simulink model "pwpf_real_signal"  (R2021b)
settings: Solver=VariableStepAuto  StartTime=0.0  StopTime=t_sim  RelTol=1e-3
values from neighbouring files (symbols this model uses):
  Km_d = inputArg(2)    [cost_pwpf_dis.m]
  scale = length_real/(max(x)-min(x))    [model3d_maker.m]
  Tm_d = inputArg(1)    [cost_pwpf_dis.m]
  u_off = inputArg(4)    [cost_pwpf.m]    (also in cost_pwpf_dis.m)
  u_on = h+u_off    [cost_pwpf.m]    (also in cost_pwpf_dis.m)
undefined symbols (not defined in the file or in its folder): min_on_off_time, sample_time
settings Model: Creator=Mehdi  LastModifiedBy=Mehdi
settings SolverCC: ZeroCrossAlgorithm=Adaptive  AlgebraicLoopSolver=TrustRegion
settings DebuggingCC: IgnoredZcDiagnostic=none  SFMachineParentedDataDiag=warning

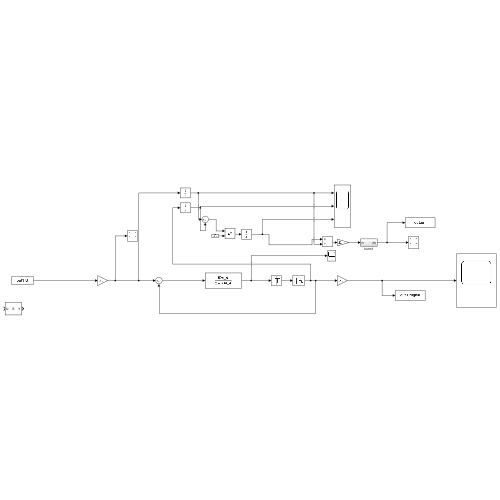
[thumbnail: Simulink's stored preview of the top-level diagram]
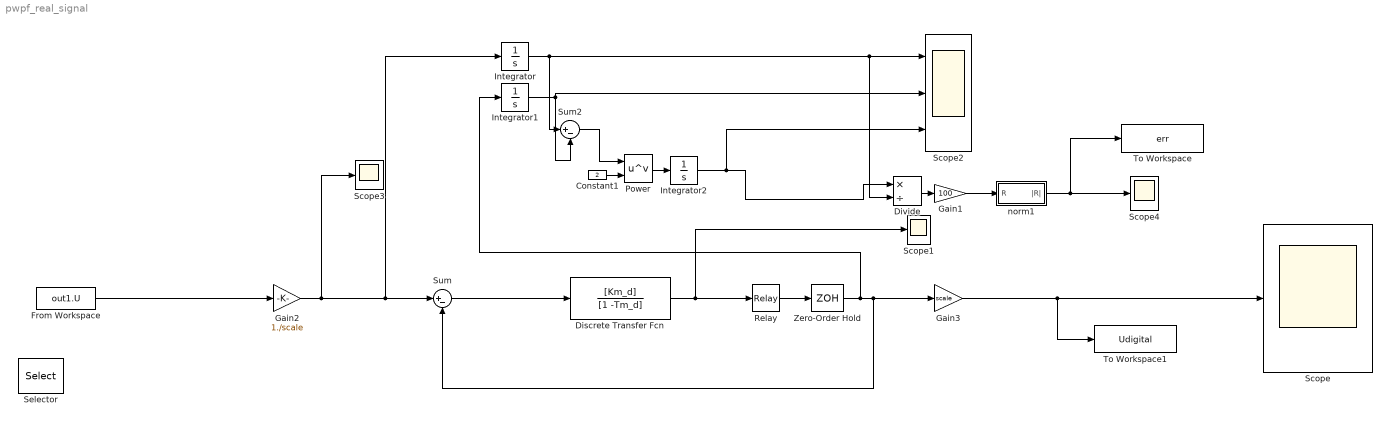
== system pwpf_real_signal ==
  Constant1 : Constant  Value=2  VectorParams1D=off
  Discrete Transfer Fcn : DiscreteTransferFcn  Numerator=[Km_d]  Denominator=[1 -Tm_d]  SampleTime=sample_time
  Divide : Product  Inputs=*/
  From Workspace : FromWorkspace  VariableName=out1.U
  Gain1 : Gain  Gain=100
  Gain2 : Gain  Gain=1./scale
  Gain3 : Gain  Gain=scale
  Integrator : Integrator
  Integrator1 : Integrator
  Integrator2 : Integrator
  Power : Math  Operator=pow  SaturateOnIntegerOverflow=on
  Relay : Relay  OnSwitchValue=u_on  OffSwitchValue=u_off  OnOutputValue=Thrust_digital
  Scope{,1,3..4} (4 alike) : Scope
  Scope2 : Scope  NumInputPorts=3
  Selector : Selector  InputPortWidth=30  IndexOptions=Index vector (dialog)  Indices=1  OutputSizes=1
  Sum : Sum  Inputs=|+-
  Sum2 : Sum  Inputs=|+-
  To Workspace : ToWorkspace  VariableName=err  SaveFormat=Timeseries  SampleTime=-1
      settings: MaxDataPoints=1
  To Workspace1 : ToWorkspace  VariableName=Udigital  SaveFormat=Timeseries  SampleTime=-1
  Zero-Order Hold : ZeroOrderHold  SampleTime=min_on_off_time
  norm1 : Subsystem
  wires:
  Discrete Transfer Fcn/1 -> Relay/1, Scope1/1
  Integrator/1 -> Sum2/1, Divide/2, Scope2/1
  Integrator1/1 -> Sum2/2, Scope2/2
  Sum2/1 -> Power/1
  Power/1 -> Integrator2/1
  Integrator2/1 -> Scope2/3, Divide/1
  Constant1/1 -> Power/2
  Relay/1 -> Zero-Order Hold/1
  Divide/1 -> Gain1/1
  Gain1/1 -> norm1/1(R)
  Sum/1 -> Discrete Transfer Fcn/1
  Zero-Order Hold/1 -> Integrator1/1, Sum/2, Gain3/1
  Gain2/1 -> Scope3/1, Integrator/1, Sum/1
  Gain3/1 -> To Workspace1/1, Scope/1
  norm1/1(|R|) -> To Workspace/1, Scope4/1
  From Workspace/1 -> Gain2/1

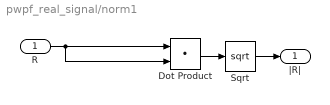
== system pwpf_real_signal/norm1 ==
  R : Inport
  Dot Product : DotProduct  InputSameDT=on  OutDataTypeStr=Inherit: Inherit via internal rule
  Sqrt : Sqrt  OutputSignalType=real  SaturateOnIntegerOverflow=on
  |R| : Outport
  wires:
  Dot Product/1 -> Sqrt/1
  R/1 -> Dot Product/1, Dot Product/2
  Sqrt/1 -> |R|/1
